simulink model "Lecture14_LSF"  (R2020b)
settings: Solver=VariableStepAuto  StartTime=0.0  StopTime=10.0  RelTol=1e-3
values from neighbouring files (symbols this model uses):
  A = [0 1; -5 -2]    [Assignment4.m]    (also in Lecture14_LSF.m = [0 1; -1 -2]; Lecture15_DigitalLSF.m = [0 1; -1 -2]; Lecture16_LSFIntegrator.m = [0 1; -1 -2]; Lecture6_3PhaseCurrent.m = 20)
  B = [0; 1]    [Assignment4.m]    (also in Lecture14_LSF.m; Lecture15_DigitalLSF.m; Lecture16_LSFIntegrator.m; dSpaceLab.m = [0; 1/La])
  C = [5 0]    [Assignment4.m]    (also in Lecture14_LSF.m = [10 0]; Lecture15_DigitalLSF.m = [10 0]; Lecture16_LSFIntegrator.m = [10 0]; dSpaceLab.m = [1, 0])
  K = 1.5    [Assignment1.m]    (also in Assignment4.m = acker(A_mark, B_mark, s_p); Lecture14_LSF.m = [1.25, 1]; Lecture15_DigitalLSF.m = acker(Ad, Bd, [z_p, z_p]); Lecture16_LSFIntegrator.m = acker(A_mark, B_mark, [s_p, s_p, s_p]))
settings Model: Creator=sebastian  LastModifiedBy=sebastian

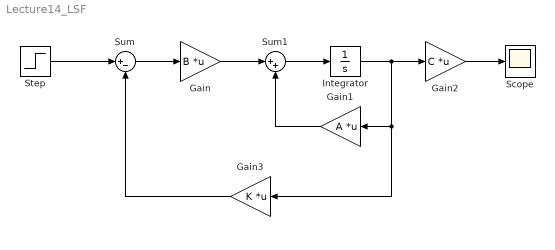
== system Lecture14_LSF ==
  Gain : Gain  Gain=B  Multiplication=Matrix(K*u)
  Gain1 : Gain  Gain=A  Multiplication=Matrix(K*u)
  Gain2 : Gain  Gain=C  Multiplication=Matrix(K*u)
  Gain3 : Gain  Gain=K  Multiplication=Matrix(K*u)
  Integrator : Integrator
  Scope : Scope
  Step : Step  SampleTime=0
  Sum : Sum  Inputs=|+-
  Sum1 : Sum  Inputs=|++
  wires:
  Step/1 -> Sum/1
  Sum/1 -> Gain/1
  Sum1/1 -> Integrator/1
  Gain/1 -> Sum1/1
  Integrator/1 -> Gain2/1, Gain3/1, Gain1/1
  Gain1/1 -> Sum1/2
  Gain3/1 -> Sum/2
  Gain2/1 -> Scope/1
